simulink model "Add_Sub_Sum"  (R2020a)
settings: Solver=VariableStepAuto  StartTime=0.0  StopTime=10.0  RelTol=1e-3
settings Model: Creator=royde  LastModifiedBy=royde

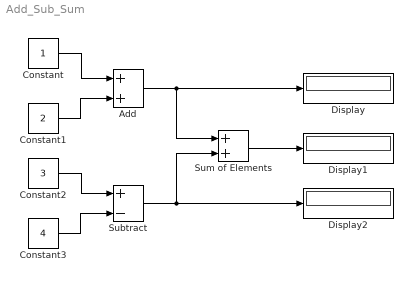
== system Add_Sub_Sum ==
  Add : Sum
  Constant : Constant
  Constant1 : Constant  Value=2
  Constant2 : Constant  Value=3
  Constant3 : Constant  Value=4
  Display : Display
  Display1 : Display
  Display2 : Display
  Subtract : Sum  Inputs=+-
  Sum of Elements : Sum
  wires:
  Constant/1 -> Add/1
  Constant1/1 -> Add/2
  Constant3/1 -> Subtract/2
  Constant2/1 -> Subtract/1
  Add/1 -> Display/1, Sum of Elements/1
  Subtract/1 -> Display2/1, Sum of Elements/2
  Sum of Elements/1 -> Display1/1
